simulink model "colas_nonlin"  (Simulink 2.09)
settings: Solver=ode45  StartTime=0.0  StopTime=50  MaxStep=1  RelTol=1e-5  AbsTol=1e-5
settings Model: SaveTime=off  SaveOutput=off  ConsistencyChecking=off  RTWTemplateMakefile=grt_unix.tmf

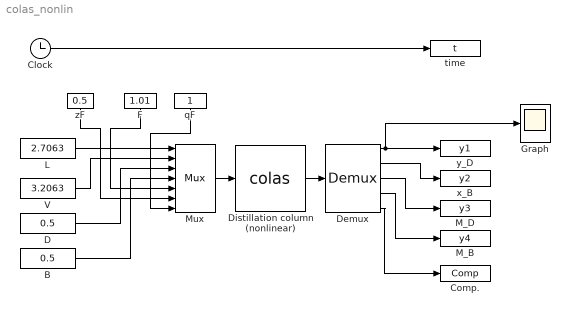
== system colas_nonlin ==
  B : Constant  Value=0.5
  Clock : Clock
  Comp. : ToWorkspace  VariableName=Comp  SampleTime=0
      settings: Buffer=1000
  D : Constant  Value=0.5
  Demux : Demux  Outputs=[1,1,1,1,41]
  Distillation column (nonlinear) : S-Function  FunctionName=colas
  F : Constant  Orientation=down  Value=1.01
  Graph : Scope
      settings: TickLabels=on  TimeRange=50  YMin=0.98  YMax=1  SaveToWorkspace=off  SaveName=ScopeData
  L : Constant  Value=2.7063
  M_B : ToWorkspace  VariableName=y4  SampleTime=0
      settings: Buffer=1000
  M_D : ToWorkspace  VariableName=y3  SampleTime=0
      settings: Buffer=1000
  Mux : Mux  Inputs=7
  V : Constant  Value=3.2063
  qF : Constant  Orientation=down  Value=1
  time : ToWorkspace  VariableName=t  SampleTime=0
      settings: Buffer=1000
  x_B : ToWorkspace  VariableName=y2  SampleTime=0
      settings: Buffer=1000
  y_D : ToWorkspace  VariableName=y1  SampleTime=0
      settings: Buffer=1000
  zF : Constant  Orientation=down  Value=0.5
  wires:
  qF/1 -> Mux/7
  Demux/1 -> Graph/1, y_D/1
  Mux/1 -> Distillation column (nonlinear)/1
  Demux/2 -> x_B/1
  Distillation column (nonlinear)/1 -> Demux/1
  Clock/1 -> time/1
  zF/1 -> Mux/6
  V/1 -> Mux/2
  F/1 -> Mux/5
  Demux/5 -> Comp./1
  Demux/4 -> M_B/1
  Demux/3 -> M_D/1
  B/1 -> Mux/4
  D/1 -> Mux/3
  L/1 -> Mux/1
